simulink model "dados"  (R2023b)
settings: Solver=VariableStepAuto  StartTime=0.0  StopTime=1000*Tpwm  RelTol=1e-3
undefined symbols (not defined in the file): A, Ae, B, Be, Tpwm, Tsim
libraries: commseqgen3 x1, spspowerguiLib x1
settings Model: Creator=luisf  LastModifiedBy=luisf

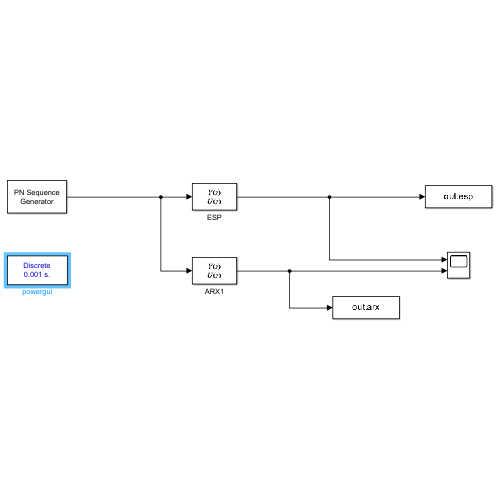
[thumbnail: Simulink's stored preview of the top-level diagram]
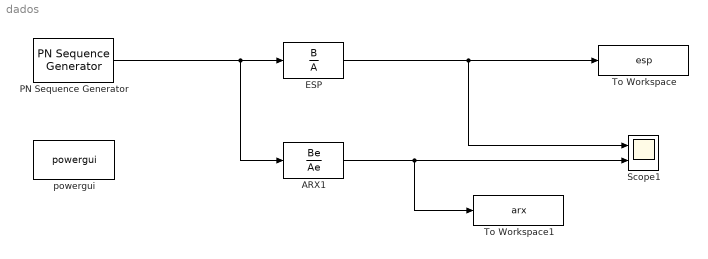
== system dados ==
  ARX1 : DiscreteTransferFcn  Numerator=Be  Denominator=Ae
  ESP : DiscreteTransferFcn  Numerator=B  Denominator=A
  PN Sequence Generator : commseqgen3/PN Sequence Generator  poly=[15 14 0]  ini_sta=ones(1, 15)  outBitMaskSource=Dialog parameter  shift=0  outVarSiz=off  maxOutSizeMode=Dialog parameter  maxOutSize=[10 1]  Ts=Tsim  sampPerFrame=1  reset=off  bitPackedOutputs=off  outDataType=double  numPackedBits=8  bitPackDataSigned=off  bitPackedOutDType=double
  Scope1 : Scope  NumInputPorts=2
  To Workspace : ToWorkspace  VariableName=esp  SampleTime=Tpwm
      settings: Save2DSignal=2-D array (concatenate along first dimension)
  To Workspace1 : ToWorkspace  VariableName=arx  SampleTime=Tpwm
      settings: Save2DSignal=2-D array (concatenate along first dimension)
  powergui : spspowerguiLib/powergui  Priority=1  SimulationMode=Discrete  SampleTime=Tpwm  frequency=60  Iterations=50  frequencyindice=60  Pbase=100e6  ErrMax=1e-4  UnitsV=kV  UnitsW=MW  buscounter=0  FunctionMessages=off  echomessages=off  EnableUseOfTLC=off  CurrentSourceSwitches=off  DisableSnubberDevices=off  DisableRonSwitches=off  DisableVfSwitches=off  DisplayEquations=off  AutomaticDiscreteSolvers=off  SolverType=Tustin/Backward Euler (TBE)  Interpol=off  ExternalGateDelay=off  methode=off  Ts=100  x0status=blocks  SPID=on  SwTol=0  HookPort=off  NonlinearTolerance=1e-4  nMaxIteration=100  ContinueOnMaxIteration=off  RestoreLinks=warning  ResistiveCurrentMeasurement=off  Frange=[0:2:500]  Ylog=off  Xlog=on  ShowGrid=off  save=off  variable=ZData  structure=0  ZoomFFT=off  StartTime=0.0  cycles=1  DisplayStyle=1  fundamental=60  FreqAxis=off  MaxFrequency=1000  frequencyindicesteady=1  RmsSteady=1  display=off
  wires:
  ESP/1 -> Scope1/1, To Workspace/1
  PN Sequence Generator/1 -> ARX1/1, ESP/1
  ARX1/1 -> To Workspace1/1, Scope1/2
